simulink library "lib_rfsoc_fec"  (R2020b)
settings: Solver=VariableStepAuto  StartTime=0.0  StopTime=10.0  RelTol=1e-3
undefined symbols (not defined in the file): d, fs, generator_polynomial
libraries: commseqgen3 x84, hdlsllib x83, $bdroot x33, simulink x22, dspsigops x13
(part 4 of 4)

== system lib_rfsoc_fec/QAM Mapping/QAM Mapping/N-Width QAM-16 Symbol Mapping Real/QAM-16 Symbol Mapping 0 ==
  bits : Inport
  Bit Slice2 : hdlsllib/Logic and Bit Operations/Bit Slice  lidx=n+3  ridx=n+2
      settings: SourceProductBaseCode=SL
  Constant1 : Constant  Value=3  OutDataTypeStr=fixdt(1,3,0)  SampleTime=-1
  Constant2 : Constant  OutDataTypeStr=fixdt(1,3,0)  SampleTime=-1
  Constant3 : Constant  Value=-1  OutDataTypeStr=fixdt(1,3,0)  SampleTime=-1
  Constant4 : Constant  Value=-3  OutDataTypeStr=fixdt(1,3,0)  SampleTime=-1
  Multiport Switch : MultiPortSwitch  DataPortOrder=Zero-based contiguous  Inputs=4  zeroidx=on
  I : Outport
  wires:
  Multiport Switch/1 -> I/1
  Constant2/1 -> Multiport Switch/5
  Constant1/1 -> Multiport Switch/4
  Constant4/1 -> Multiport Switch/2
  Constant3/1 -> Multiport Switch/3
  bits/1 -> Bit Slice2/1
  Bit Slice2/1 -> Multiport Switch/1

== system lib_rfsoc_fec/QAM Mapping/QAM Mapping/N-Width QAM-16 Symbol Mapping Real/QAM-16 Symbol Mapping 1 ==
  bits : Inport
  Bit Slice2 : hdlsllib/Logic and Bit Operations/Bit Slice  lidx=n+3  ridx=n+2
      settings: SourceProductBaseCode=SL
  Constant1 : Constant  Value=3  OutDataTypeStr=fixdt(1,3,0)  SampleTime=-1
  Constant2 : Constant  OutDataTypeStr=fixdt(1,3,0)  SampleTime=-1
  Constant3 : Constant  Value=-1  OutDataTypeStr=fixdt(1,3,0)  SampleTime=-1
  Constant4 : Constant  Value=-3  OutDataTypeStr=fixdt(1,3,0)  SampleTime=-1
  Multiport Switch : MultiPortSwitch  DataPortOrder=Zero-based contiguous  Inputs=4  zeroidx=on
  I : Outport
  wires:
  Bit Slice2/1 -> Multiport Switch/1
  bits/1 -> Bit Slice2/1
  Constant3/1 -> Multiport Switch/3
  Constant4/1 -> Multiport Switch/2
  Constant1/1 -> Multiport Switch/4
  Constant2/1 -> Multiport Switch/5
  Multiport Switch/1 -> I/1

== system lib_rfsoc_fec/QAM Mapping/QAM Mapping/N-Width QAM-16 Symbol Mapping Real/QAM-16 Symbol Mapping 10 ==
  bits : Inport
  Bit Slice2 : hdlsllib/Logic and Bit Operations/Bit Slice  lidx=n+3  ridx=n+2
      settings: SourceProductBaseCode=SL
  Constant1 : Constant  Value=3  OutDataTypeStr=fixdt(1,3,0)  SampleTime=-1
  Constant2 : Constant  OutDataTypeStr=fixdt(1,3,0)  SampleTime=-1
  Constant3 : Constant  Value=-1  OutDataTypeStr=fixdt(1,3,0)  SampleTime=-1
  Constant4 : Constant  Value=-3  OutDataTypeStr=fixdt(1,3,0)  SampleTime=-1
  Multiport Switch : MultiPortSwitch  DataPortOrder=Zero-based contiguous  Inputs=4  zeroidx=on
  I : Outport
  wires:
  Bit Slice2/1 -> Multiport Switch/1
  bits/1 -> Bit Slice2/1
  Constant3/1 -> Multiport Switch/3
  Constant4/1 -> Multiport Switch/2
  Constant1/1 -> Multiport Switch/4
  Constant2/1 -> Multiport Switch/5
  Multiport Switch/1 -> I/1

== system lib_rfsoc_fec/QAM Mapping/QAM Mapping/N-Width QAM-16 Symbol Mapping Real/QAM-16 Symbol Mapping 11 ==
  bits : Inport
  Bit Slice2 : hdlsllib/Logic and Bit Operations/Bit Slice  lidx=n+3  ridx=n+2
      settings: SourceProductBaseCode=SL
  Constant1 : Constant  Value=3  OutDataTypeStr=fixdt(1,3,0)  SampleTime=-1
  Constant2 : Constant  OutDataTypeStr=fixdt(1,3,0)  SampleTime=-1
  Constant3 : Constant  Value=-1  OutDataTypeStr=fixdt(1,3,0)  SampleTime=-1
  Constant4 : Constant  Value=-3  OutDataTypeStr=fixdt(1,3,0)  SampleTime=-1
  Multiport Switch : MultiPortSwitch  DataPortOrder=Zero-based contiguous  Inputs=4  zeroidx=on
  I : Outport
  wires:
  Bit Slice2/1 -> Multiport Switch/1
  bits/1 -> Bit Slice2/1
  Constant3/1 -> Multiport Switch/3
  Constant4/1 -> Multiport Switch/2
  Constant1/1 -> Multiport Switch/4
  Constant2/1 -> Multiport Switch/5
  Multiport Switch/1 -> I/1

== system lib_rfsoc_fec/QAM Mapping/QAM Mapping/N-Width QAM-16 Symbol Mapping Real/QAM-16 Symbol Mapping 12 ==
  bits : Inport
  Bit Slice2 : hdlsllib/Logic and Bit Operations/Bit Slice  lidx=n+3  ridx=n+2
      settings: SourceProductBaseCode=SL
  Constant1 : Constant  Value=3  OutDataTypeStr=fixdt(1,3,0)  SampleTime=-1
  Constant2 : Constant  OutDataTypeStr=fixdt(1,3,0)  SampleTime=-1
  Constant3 : Constant  Value=-1  OutDataTypeStr=fixdt(1,3,0)  SampleTime=-1
  Constant4 : Constant  Value=-3  OutDataTypeStr=fixdt(1,3,0)  SampleTime=-1
  Multiport Switch : MultiPortSwitch  DataPortOrder=Zero-based contiguous  Inputs=4  zeroidx=on
  I : Outport
  wires:
  Bit Slice2/1 -> Multiport Switch/1
  bits/1 -> Bit Slice2/1
  Constant3/1 -> Multiport Switch/3
  Constant4/1 -> Multiport Switch/2
  Constant1/1 -> Multiport Switch/4
  Constant2/1 -> Multiport Switch/5
  Multiport Switch/1 -> I/1

== system lib_rfsoc_fec/QAM Mapping/QAM Mapping/N-Width QAM-16 Symbol Mapping Real/QAM-16 Symbol Mapping 13 ==
  bits : Inport
  Bit Slice2 : hdlsllib/Logic and Bit Operations/Bit Slice  lidx=n+3  ridx=n+2
      settings: SourceProductBaseCode=SL
  Constant1 : Constant  Value=3  OutDataTypeStr=fixdt(1,3,0)  SampleTime=-1
  Constant2 : Constant  OutDataTypeStr=fixdt(1,3,0)  SampleTime=-1
  Constant3 : Constant  Value=-1  OutDataTypeStr=fixdt(1,3,0)  SampleTime=-1
  Constant4 : Constant  Value=-3  OutDataTypeStr=fixdt(1,3,0)  SampleTime=-1
  Multiport Switch : MultiPortSwitch  DataPortOrder=Zero-based contiguous  Inputs=4  zeroidx=on
  I : Outport
  wires:
  Bit Slice2/1 -> Multiport Switch/1
  bits/1 -> Bit Slice2/1
  Constant3/1 -> Multiport Switch/3
  Constant4/1 -> Multiport Switch/2
  Constant1/1 -> Multiport Switch/4
  Constant2/1 -> Multiport Switch/5
  Multiport Switch/1 -> I/1

== system lib_rfsoc_fec/QAM Mapping/QAM Mapping/N-Width QAM-16 Symbol Mapping Real/QAM-16 Symbol Mapping 14 ==
  bits : Inport
  Bit Slice2 : hdlsllib/Logic and Bit Operations/Bit Slice  lidx=n+3  ridx=n+2
      settings: SourceProductBaseCode=SL
  Constant1 : Constant  Value=3  OutDataTypeStr=fixdt(1,3,0)  SampleTime=-1
  Constant2 : Constant  OutDataTypeStr=fixdt(1,3,0)  SampleTime=-1
  Constant3 : Constant  Value=-1  OutDataTypeStr=fixdt(1,3,0)  SampleTime=-1
  Constant4 : Constant  Value=-3  OutDataTypeStr=fixdt(1,3,0)  SampleTime=-1
  Multiport Switch : MultiPortSwitch  DataPortOrder=Zero-based contiguous  Inputs=4  zeroidx=on
  I : Outport
  wires:
  Bit Slice2/1 -> Multiport Switch/1
  bits/1 -> Bit Slice2/1
  Constant3/1 -> Multiport Switch/3
  Constant4/1 -> Multiport Switch/2
  Constant1/1 -> Multiport Switch/4
  Constant2/1 -> Multiport Switch/5
  Multiport Switch/1 -> I/1

== system lib_rfsoc_fec/QAM Mapping/QAM Mapping/N-Width QAM-16 Symbol Mapping Real/QAM-16 Symbol Mapping 15 ==
  bits : Inport
  Bit Slice2 : hdlsllib/Logic and Bit Operations/Bit Slice  lidx=n+3  ridx=n+2
      settings: SourceProductBaseCode=SL
  Constant1 : Constant  Value=3  OutDataTypeStr=fixdt(1,3,0)  SampleTime=-1
  Constant2 : Constant  OutDataTypeStr=fixdt(1,3,0)  SampleTime=-1
  Constant3 : Constant  Value=-1  OutDataTypeStr=fixdt(1,3,0)  SampleTime=-1
  Constant4 : Constant  Value=-3  OutDataTypeStr=fixdt(1,3,0)  SampleTime=-1
  Multiport Switch : MultiPortSwitch  DataPortOrder=Zero-based contiguous  Inputs=4  zeroidx=on
  I : Outport
  wires:
  Bit Slice2/1 -> Multiport Switch/1
  bits/1 -> Bit Slice2/1
  Constant3/1 -> Multiport Switch/3
  Constant4/1 -> Multiport Switch/2
  Constant1/1 -> Multiport Switch/4
  Constant2/1 -> Multiport Switch/5
  Multiport Switch/1 -> I/1

== system lib_rfsoc_fec/QAM Mapping/QAM Mapping/N-Width QAM-16 Symbol Mapping Real/QAM-16 Symbol Mapping 16 ==
  bits : Inport
  Bit Slice2 : hdlsllib/Logic and Bit Operations/Bit Slice  lidx=n+3  ridx=n+2
      settings: SourceProductBaseCode=SL
  Constant1 : Constant  Value=3  OutDataTypeStr=fixdt(1,3,0)  SampleTime=-1
  Constant2 : Constant  OutDataTypeStr=fixdt(1,3,0)  SampleTime=-1
  Constant3 : Constant  Value=-1  OutDataTypeStr=fixdt(1,3,0)  SampleTime=-1
  Constant4 : Constant  Value=-3  OutDataTypeStr=fixdt(1,3,0)  SampleTime=-1
  Multiport Switch : MultiPortSwitch  DataPortOrder=Zero-based contiguous  Inputs=4  zeroidx=on
  I : Outport
  wires:
  Bit Slice2/1 -> Multiport Switch/1
  bits/1 -> Bit Slice2/1
  Constant3/1 -> Multiport Switch/3
  Constant4/1 -> Multiport Switch/2
  Constant1/1 -> Multiport Switch/4
  Constant2/1 -> Multiport Switch/5
  Multiport Switch/1 -> I/1

== system lib_rfsoc_fec/QAM Mapping/QAM Mapping/N-Width QAM-16 Symbol Mapping Real/QAM-16 Symbol Mapping 17 ==
  bits : Inport
  Bit Slice2 : hdlsllib/Logic and Bit Operations/Bit Slice  lidx=n+3  ridx=n+2
      settings: SourceProductBaseCode=SL
  Constant1 : Constant  Value=3  OutDataTypeStr=fixdt(1,3,0)  SampleTime=-1
  Constant2 : Constant  OutDataTypeStr=fixdt(1,3,0)  SampleTime=-1
  Constant3 : Constant  Value=-1  OutDataTypeStr=fixdt(1,3,0)  SampleTime=-1
  Constant4 : Constant  Value=-3  OutDataTypeStr=fixdt(1,3,0)  SampleTime=-1
  Multiport Switch : MultiPortSwitch  DataPortOrder=Zero-based contiguous  Inputs=4  zeroidx=on
  I : Outport
  wires:
  Bit Slice2/1 -> Multiport Switch/1
  bits/1 -> Bit Slice2/1
  Constant3/1 -> Multiport Switch/3
  Constant4/1 -> Multiport Switch/2
  Constant1/1 -> Multiport Switch/4
  Constant2/1 -> Multiport Switch/5
  Multiport Switch/1 -> I/1

== system lib_rfsoc_fec/QAM Mapping/QAM Mapping/N-Width QAM-16 Symbol Mapping Real/QAM-16 Symbol Mapping 18 ==
  bits : Inport
  Bit Slice2 : hdlsllib/Logic and Bit Operations/Bit Slice  lidx=n+3  ridx=n+2
      settings: SourceProductBaseCode=SL
  Constant1 : Constant  Value=3  OutDataTypeStr=fixdt(1,3,0)  SampleTime=-1
  Constant2 : Constant  OutDataTypeStr=fixdt(1,3,0)  SampleTime=-1
  Constant3 : Constant  Value=-1  OutDataTypeStr=fixdt(1,3,0)  SampleTime=-1
  Constant4 : Constant  Value=-3  OutDataTypeStr=fixdt(1,3,0)  SampleTime=-1
  Multiport Switch : MultiPortSwitch  DataPortOrder=Zero-based contiguous  Inputs=4  zeroidx=on
  I : Outport
  wires:
  Bit Slice2/1 -> Multiport Switch/1
  bits/1 -> Bit Slice2/1
  Constant3/1 -> Multiport Switch/3
  Constant4/1 -> Multiport Switch/2
  Constant1/1 -> Multiport Switch/4
  Constant2/1 -> Multiport Switch/5
  Multiport Switch/1 -> I/1

== system lib_rfsoc_fec/QAM Mapping/QAM Mapping/N-Width QAM-16 Symbol Mapping Real/QAM-16 Symbol Mapping 19 ==
  bits : Inport
  Bit Slice2 : hdlsllib/Logic and Bit Operations/Bit Slice  lidx=n+3  ridx=n+2
      settings: SourceProductBaseCode=SL
  Constant1 : Constant  Value=3  OutDataTypeStr=fixdt(1,3,0)  SampleTime=-1
  Constant2 : Constant  OutDataTypeStr=fixdt(1,3,0)  SampleTime=-1
  Constant3 : Constant  Value=-1  OutDataTypeStr=fixdt(1,3,0)  SampleTime=-1
  Constant4 : Constant  Value=-3  OutDataTypeStr=fixdt(1,3,0)  SampleTime=-1
  Multiport Switch : MultiPortSwitch  DataPortOrder=Zero-based contiguous  Inputs=4  zeroidx=on
  I : Outport
  wires:
  Bit Slice2/1 -> Multiport Switch/1
  bits/1 -> Bit Slice2/1
  Constant3/1 -> Multiport Switch/3
  Constant4/1 -> Multiport Switch/2
  Constant1/1 -> Multiport Switch/4
  Constant2/1 -> Multiport Switch/5
  Multiport Switch/1 -> I/1

== system lib_rfsoc_fec/QAM Mapping/QAM Mapping/N-Width QAM-16 Symbol Mapping Real/QAM-16 Symbol Mapping 2 ==
  bits : Inport
  Bit Slice2 : hdlsllib/Logic and Bit Operations/Bit Slice  lidx=n+3  ridx=n+2
      settings: SourceProductBaseCode=SL
  Constant1 : Constant  Value=3  OutDataTypeStr=fixdt(1,3,0)  SampleTime=-1
  Constant2 : Constant  OutDataTypeStr=fixdt(1,3,0)  SampleTime=-1
  Constant3 : Constant  Value=-1  OutDataTypeStr=fixdt(1,3,0)  SampleTime=-1
  Constant4 : Constant  Value=-3  OutDataTypeStr=fixdt(1,3,0)  SampleTime=-1
  Multiport Switch : MultiPortSwitch  DataPortOrder=Zero-based contiguous  Inputs=4  zeroidx=on
  I : Outport
  wires:
  Bit Slice2/1 -> Multiport Switch/1
  bits/1 -> Bit Slice2/1
  Constant3/1 -> Multiport Switch/3
  Constant4/1 -> Multiport Switch/2
  Constant1/1 -> Multiport Switch/4
  Constant2/1 -> Multiport Switch/5
  Multiport Switch/1 -> I/1

== system lib_rfsoc_fec/QAM Mapping/QAM Mapping/N-Width QAM-16 Symbol Mapping Real/QAM-16 Symbol Mapping 20 ==
  bits : Inport
  Bit Slice2 : hdlsllib/Logic and Bit Operations/Bit Slice  lidx=n+3  ridx=n+2
      settings: SourceProductBaseCode=SL
  Constant1 : Constant  Value=3  OutDataTypeStr=fixdt(1,3,0)  SampleTime=-1
  Constant2 : Constant  OutDataTypeStr=fixdt(1,3,0)  SampleTime=-1
  Constant3 : Constant  Value=-1  OutDataTypeStr=fixdt(1,3,0)  SampleTime=-1
  Constant4 : Constant  Value=-3  OutDataTypeStr=fixdt(1,3,0)  SampleTime=-1
  Multiport Switch : MultiPortSwitch  DataPortOrder=Zero-based contiguous  Inputs=4  zeroidx=on
  I : Outport
  wires:
  Bit Slice2/1 -> Multiport Switch/1
  bits/1 -> Bit Slice2/1
  Constant3/1 -> Multiport Switch/3
  Constant4/1 -> Multiport Switch/2
  Constant1/1 -> Multiport Switch/4
  Constant2/1 -> Multiport Switch/5
  Multiport Switch/1 -> I/1

== system lib_rfsoc_fec/QAM Mapping/QAM Mapping/N-Width QAM-16 Symbol Mapping Real/QAM-16 Symbol Mapping 21 ==
  bits : Inport
  Bit Slice2 : hdlsllib/Logic and Bit Operations/Bit Slice  lidx=n+3  ridx=n+2
      settings: SourceProductBaseCode=SL
  Constant1 : Constant  Value=3  OutDataTypeStr=fixdt(1,3,0)  SampleTime=-1
  Constant2 : Constant  OutDataTypeStr=fixdt(1,3,0)  SampleTime=-1
  Constant3 : Constant  Value=-1  OutDataTypeStr=fixdt(1,3,0)  SampleTime=-1
  Constant4 : Constant  Value=-3  OutDataTypeStr=fixdt(1,3,0)  SampleTime=-1
  Multiport Switch : MultiPortSwitch  DataPortOrder=Zero-based contiguous  Inputs=4  zeroidx=on
  I : Outport
  wires:
  Bit Slice2/1 -> Multiport Switch/1
  bits/1 -> Bit Slice2/1
  Constant3/1 -> Multiport Switch/3
  Constant4/1 -> Multiport Switch/2
  Constant1/1 -> Multiport Switch/4
  Constant2/1 -> Multiport Switch/5
  Multiport Switch/1 -> I/1

== system lib_rfsoc_fec/QAM Mapping/QAM Mapping/N-Width QAM-16 Symbol Mapping Real/QAM-16 Symbol Mapping 22 ==
  bits : Inport
  Bit Slice2 : hdlsllib/Logic and Bit Operations/Bit Slice  lidx=n+3  ridx=n+2
      settings: SourceProductBaseCode=SL
  Constant1 : Constant  Value=3  OutDataTypeStr=fixdt(1,3,0)  SampleTime=-1
  Constant2 : Constant  OutDataTypeStr=fixdt(1,3,0)  SampleTime=-1
  Constant3 : Constant  Value=-1  OutDataTypeStr=fixdt(1,3,0)  SampleTime=-1
  Constant4 : Constant  Value=-3  OutDataTypeStr=fixdt(1,3,0)  SampleTime=-1
  Multiport Switch : MultiPortSwitch  DataPortOrder=Zero-based contiguous  Inputs=4  zeroidx=on
  I : Outport
  wires:
  Bit Slice2/1 -> Multiport Switch/1
  bits/1 -> Bit Slice2/1
  Constant3/1 -> Multiport Switch/3
  Constant4/1 -> Multiport Switch/2
  Constant1/1 -> Multiport Switch/4
  Constant2/1 -> Multiport Switch/5
  Multiport Switch/1 -> I/1

== system lib_rfsoc_fec/QAM Mapping/QAM Mapping/N-Width QAM-16 Symbol Mapping Real/QAM-16 Symbol Mapping 23 ==
  bits : Inport
  Bit Slice2 : hdlsllib/Logic and Bit Operations/Bit Slice  lidx=n+3  ridx=n+2
      settings: SourceProductBaseCode=SL
  Constant1 : Constant  Value=3  OutDataTypeStr=fixdt(1,3,0)  SampleTime=-1
  Constant2 : Constant  OutDataTypeStr=fixdt(1,3,0)  SampleTime=-1
  Constant3 : Constant  Value=-1  OutDataTypeStr=fixdt(1,3,0)  SampleTime=-1
  Constant4 : Constant  Value=-3  OutDataTypeStr=fixdt(1,3,0)  SampleTime=-1
  Multiport Switch : MultiPortSwitch  DataPortOrder=Zero-based contiguous  Inputs=4  zeroidx=on
  I : Outport
  wires:
  Bit Slice2/1 -> Multiport Switch/1
  bits/1 -> Bit Slice2/1
  Constant3/1 -> Multiport Switch/3
  Constant4/1 -> Multiport Switch/2
  Constant1/1 -> Multiport Switch/4
  Constant2/1 -> Multiport Switch/5
  Multiport Switch/1 -> I/1

== system lib_rfsoc_fec/QAM Mapping/QAM Mapping/N-Width QAM-16 Symbol Mapping Real/QAM-16 Symbol Mapping 24 ==
  bits : Inport
  Bit Slice2 : hdlsllib/Logic and Bit Operations/Bit Slice  lidx=n+3  ridx=n+2
      settings: SourceProductBaseCode=SL
  Constant1 : Constant  Value=3  OutDataTypeStr=fixdt(1,3,0)  SampleTime=-1
  Constant2 : Constant  OutDataTypeStr=fixdt(1,3,0)  SampleTime=-1
  Constant3 : Constant  Value=-1  OutDataTypeStr=fixdt(1,3,0)  SampleTime=-1
  Constant4 : Constant  Value=-3  OutDataTypeStr=fixdt(1,3,0)  SampleTime=-1
  Multiport Switch : MultiPortSwitch  DataPortOrder=Zero-based contiguous  Inputs=4  zeroidx=on
  I : Outport
  wires:
  Bit Slice2/1 -> Multiport Switch/1
  bits/1 -> Bit Slice2/1
  Constant3/1 -> Multiport Switch/3
  Constant4/1 -> Multiport Switch/2
  Constant1/1 -> Multiport Switch/4
  Constant2/1 -> Multiport Switch/5
  Multiport Switch/1 -> I/1

== system lib_rfsoc_fec/QAM Mapping/QAM Mapping/N-Width QAM-16 Symbol Mapping Real/QAM-16 Symbol Mapping 25 ==
  bits : Inport
  Bit Slice2 : hdlsllib/Logic and Bit Operations/Bit Slice  lidx=n+3  ridx=n+2
      settings: SourceProductBaseCode=SL
  Constant1 : Constant  Value=3  OutDataTypeStr=fixdt(1,3,0)  SampleTime=-1
  Constant2 : Constant  OutDataTypeStr=fixdt(1,3,0)  SampleTime=-1
  Constant3 : Constant  Value=-1  OutDataTypeStr=fixdt(1,3,0)  SampleTime=-1
  Constant4 : Constant  Value=-3  OutDataTypeStr=fixdt(1,3,0)  SampleTime=-1
  Multiport Switch : MultiPortSwitch  DataPortOrder=Zero-based contiguous  Inputs=4  zeroidx=on
  I : Outport
  wires:
  Bit Slice2/1 -> Multiport Switch/1
  bits/1 -> Bit Slice2/1
  Constant3/1 -> Multiport Switch/3
  Constant4/1 -> Multiport Switch/2
  Constant1/1 -> Multiport Switch/4
  Constant2/1 -> Multiport Switch/5
  Multiport Switch/1 -> I/1

== system lib_rfsoc_fec/QAM Mapping/QAM Mapping/N-Width QAM-16 Symbol Mapping Real/QAM-16 Symbol Mapping 26 ==
  bits : Inport
  Bit Slice2 : hdlsllib/Logic and Bit Operations/Bit Slice  lidx=n+3  ridx=n+2
      settings: SourceProductBaseCode=SL
  Constant1 : Constant  Value=3  OutDataTypeStr=fixdt(1,3,0)  SampleTime=-1
  Constant2 : Constant  OutDataTypeStr=fixdt(1,3,0)  SampleTime=-1
  Constant3 : Constant  Value=-1  OutDataTypeStr=fixdt(1,3,0)  SampleTime=-1
  Constant4 : Constant  Value=-3  OutDataTypeStr=fixdt(1,3,0)  SampleTime=-1
  Multiport Switch : MultiPortSwitch  DataPortOrder=Zero-based contiguous  Inputs=4  zeroidx=on
  I : Outport
  wires:
  Bit Slice2/1 -> Multiport Switch/1
  bits/1 -> Bit Slice2/1
  Constant3/1 -> Multiport Switch/3
  Constant4/1 -> Multiport Switch/2
  Constant1/1 -> Multiport Switch/4
  Constant2/1 -> Multiport Switch/5
  Multiport Switch/1 -> I/1

== system lib_rfsoc_fec/QAM Mapping/QAM Mapping/N-Width QAM-16 Symbol Mapping Real/QAM-16 Symbol Mapping 27 ==
  bits : Inport
  Bit Slice2 : hdlsllib/Logic and Bit Operations/Bit Slice  lidx=n+3  ridx=n+2
      settings: SourceProductBaseCode=SL
  Constant1 : Constant  Value=3  OutDataTypeStr=fixdt(1,3,0)  SampleTime=-1
  Constant2 : Constant  OutDataTypeStr=fixdt(1,3,0)  SampleTime=-1
  Constant3 : Constant  Value=-1  OutDataTypeStr=fixdt(1,3,0)  SampleTime=-1
  Constant4 : Constant  Value=-3  OutDataTypeStr=fixdt(1,3,0)  SampleTime=-1
  Multiport Switch : MultiPortSwitch  DataPortOrder=Zero-based contiguous  Inputs=4  zeroidx=on
  I : Outport
  wires:
  Bit Slice2/1 -> Multiport Switch/1
  bits/1 -> Bit Slice2/1
  Constant3/1 -> Multiport Switch/3
  Constant4/1 -> Multiport Switch/2
  Constant1/1 -> Multiport Switch/4
  Constant2/1 -> Multiport Switch/5
  Multiport Switch/1 -> I/1

== system lib_rfsoc_fec/QAM Mapping/QAM Mapping/N-Width QAM-16 Symbol Mapping Real/QAM-16 Symbol Mapping 28 ==
  bits : Inport
  Bit Slice2 : hdlsllib/Logic and Bit Operations/Bit Slice  lidx=n+3  ridx=n+2
      settings: SourceProductBaseCode=SL
  Constant1 : Constant  Value=3  OutDataTypeStr=fixdt(1,3,0)  SampleTime=-1
  Constant2 : Constant  OutDataTypeStr=fixdt(1,3,0)  SampleTime=-1
  Constant3 : Constant  Value=-1  OutDataTypeStr=fixdt(1,3,0)  SampleTime=-1
  Constant4 : Constant  Value=-3  OutDataTypeStr=fixdt(1,3,0)  SampleTime=-1
  Multiport Switch : MultiPortSwitch  DataPortOrder=Zero-based contiguous  Inputs=4  zeroidx=on
  I : Outport
  wires:
  Bit Slice2/1 -> Multiport Switch/1
  bits/1 -> Bit Slice2/1
  Constant3/1 -> Multiport Switch/3
  Constant4/1 -> Multiport Switch/2
  Constant1/1 -> Multiport Switch/4
  Constant2/1 -> Multiport Switch/5
  Multiport Switch/1 -> I/1

== system lib_rfsoc_fec/QAM Mapping/QAM Mapping/N-Width QAM-16 Symbol Mapping Real/QAM-16 Symbol Mapping 29 ==
  bits : Inport
  Bit Slice2 : hdlsllib/Logic and Bit Operations/Bit Slice  lidx=n+3  ridx=n+2
      settings: SourceProductBaseCode=SL
  Constant1 : Constant  Value=3  OutDataTypeStr=fixdt(1,3,0)  SampleTime=-1
  Constant2 : Constant  OutDataTypeStr=fixdt(1,3,0)  SampleTime=-1
  Constant3 : Constant  Value=-1  OutDataTypeStr=fixdt(1,3,0)  SampleTime=-1
  Constant4 : Constant  Value=-3  OutDataTypeStr=fixdt(1,3,0)  SampleTime=-1
  Multiport Switch : MultiPortSwitch  DataPortOrder=Zero-based contiguous  Inputs=4  zeroidx=on
  I : Outport
  wires:
  Bit Slice2/1 -> Multiport Switch/1
  bits/1 -> Bit Slice2/1
  Constant3/1 -> Multiport Switch/3
  Constant4/1 -> Multiport Switch/2
  Constant1/1 -> Multiport Switch/4
  Constant2/1 -> Multiport Switch/5
  Multiport Switch/1 -> I/1

== system lib_rfsoc_fec/QAM Mapping/QAM Mapping/N-Width QAM-16 Symbol Mapping Real/QAM-16 Symbol Mapping 3 ==
  bits : Inport
  Bit Slice2 : hdlsllib/Logic and Bit Operations/Bit Slice  lidx=n+3  ridx=n+2
      settings: SourceProductBaseCode=SL
  Constant1 : Constant  Value=3  OutDataTypeStr=fixdt(1,3,0)  SampleTime=-1
  Constant2 : Constant  OutDataTypeStr=fixdt(1,3,0)  SampleTime=-1
  Constant3 : Constant  Value=-1  OutDataTypeStr=fixdt(1,3,0)  SampleTime=-1
  Constant4 : Constant  Value=-3  OutDataTypeStr=fixdt(1,3,0)  SampleTime=-1
  Multiport Switch : MultiPortSwitch  DataPortOrder=Zero-based contiguous  Inputs=4  zeroidx=on
  I : Outport
  wires:
  Bit Slice2/1 -> Multiport Switch/1
  bits/1 -> Bit Slice2/1
  Constant3/1 -> Multiport Switch/3
  Constant4/1 -> Multiport Switch/2
  Constant1/1 -> Multiport Switch/4
  Constant2/1 -> Multiport Switch/5
  Multiport Switch/1 -> I/1

== system lib_rfsoc_fec/QAM Mapping/QAM Mapping/N-Width QAM-16 Symbol Mapping Real/QAM-16 Symbol Mapping 30 ==
  bits : Inport
  Bit Slice2 : hdlsllib/Logic and Bit Operations/Bit Slice  lidx=n+3  ridx=n+2
      settings: SourceProductBaseCode=SL
  Constant1 : Constant  Value=3  OutDataTypeStr=fixdt(1,3,0)  SampleTime=-1
  Constant2 : Constant  OutDataTypeStr=fixdt(1,3,0)  SampleTime=-1
  Constant3 : Constant  Value=-1  OutDataTypeStr=fixdt(1,3,0)  SampleTime=-1
  Constant4 : Constant  Value=-3  OutDataTypeStr=fixdt(1,3,0)  SampleTime=-1
  Multiport Switch : MultiPortSwitch  DataPortOrder=Zero-based contiguous  Inputs=4  zeroidx=on
  I : Outport
  wires:
  Bit Slice2/1 -> Multiport Switch/1
  bits/1 -> Bit Slice2/1
  Constant3/1 -> Multiport Switch/3
  Constant4/1 -> Multiport Switch/2
  Constant1/1 -> Multiport Switch/4
  Constant2/1 -> Multiport Switch/5
  Multiport Switch/1 -> I/1

== system lib_rfsoc_fec/QAM Mapping/QAM Mapping/N-Width QAM-16 Symbol Mapping Real/QAM-16 Symbol Mapping 31 ==
  bits : Inport
  Bit Slice2 : hdlsllib/Logic and Bit Operations/Bit Slice  lidx=n+3  ridx=n+2
      settings: SourceProductBaseCode=SL
  Constant1 : Constant  Value=3  OutDataTypeStr=fixdt(1,3,0)  SampleTime=-1
  Constant2 : Constant  OutDataTypeStr=fixdt(1,3,0)  SampleTime=-1
  Constant3 : Constant  Value=-1  OutDataTypeStr=fixdt(1,3,0)  SampleTime=-1
  Constant4 : Constant  Value=-3  OutDataTypeStr=fixdt(1,3,0)  SampleTime=-1
  Multiport Switch : MultiPortSwitch  DataPortOrder=Zero-based contiguous  Inputs=4  zeroidx=on
  I : Outport
  wires:
  Bit Slice2/1 -> Multiport Switch/1
  bits/1 -> Bit Slice2/1
  Constant3/1 -> Multiport Switch/3
  Constant4/1 -> Multiport Switch/2
  Constant1/1 -> Multiport Switch/4
  Constant2/1 -> Multiport Switch/5
  Multiport Switch/1 -> I/1

== system lib_rfsoc_fec/QAM Mapping/QAM Mapping/N-Width QAM-16 Symbol Mapping Real/QAM-16 Symbol Mapping 4 ==
  bits : Inport
  Bit Slice2 : hdlsllib/Logic and Bit Operations/Bit Slice  lidx=n+3  ridx=n+2
      settings: SourceProductBaseCode=SL
  Constant1 : Constant  Value=3  OutDataTypeStr=fixdt(1,3,0)  SampleTime=-1
  Constant2 : Constant  OutDataTypeStr=fixdt(1,3,0)  SampleTime=-1
  Constant3 : Constant  Value=-1  OutDataTypeStr=fixdt(1,3,0)  SampleTime=-1
  Constant4 : Constant  Value=-3  OutDataTypeStr=fixdt(1,3,0)  SampleTime=-1
  Multiport Switch : MultiPortSwitch  DataPortOrder=Zero-based contiguous  Inputs=4  zeroidx=on
  I : Outport
  wires:
  Bit Slice2/1 -> Multiport Switch/1
  bits/1 -> Bit Slice2/1
  Constant3/1 -> Multiport Switch/3
  Constant4/1 -> Multiport Switch/2
  Constant1/1 -> Multiport Switch/4
  Constant2/1 -> Multiport Switch/5
  Multiport Switch/1 -> I/1

== system lib_rfsoc_fec/QAM Mapping/QAM Mapping/N-Width QAM-16 Symbol Mapping Real/QAM-16 Symbol Mapping 5 ==
  bits : Inport
  Bit Slice2 : hdlsllib/Logic and Bit Operations/Bit Slice  lidx=n+3  ridx=n+2
      settings: SourceProductBaseCode=SL
  Constant1 : Constant  Value=3  OutDataTypeStr=fixdt(1,3,0)  SampleTime=-1
  Constant2 : Constant  OutDataTypeStr=fixdt(1,3,0)  SampleTime=-1
  Constant3 : Constant  Value=-1  OutDataTypeStr=fixdt(1,3,0)  SampleTime=-1
  Constant4 : Constant  Value=-3  OutDataTypeStr=fixdt(1,3,0)  SampleTime=-1
  Multiport Switch : MultiPortSwitch  DataPortOrder=Zero-based contiguous  Inputs=4  zeroidx=on
  I : Outport
  wires:
  Bit Slice2/1 -> Multiport Switch/1
  bits/1 -> Bit Slice2/1
  Constant3/1 -> Multiport Switch/3
  Constant4/1 -> Multiport Switch/2
  Constant1/1 -> Multiport Switch/4
  Constant2/1 -> Multiport Switch/5
  Multiport Switch/1 -> I/1

== system lib_rfsoc_fec/QAM Mapping/QAM Mapping/N-Width QAM-16 Symbol Mapping Real/QAM-16 Symbol Mapping 6 ==
  bits : Inport
  Bit Slice2 : hdlsllib/Logic and Bit Operations/Bit Slice  lidx=n+3  ridx=n+2
      settings: SourceProductBaseCode=SL
  Constant1 : Constant  Value=3  OutDataTypeStr=fixdt(1,3,0)  SampleTime=-1
  Constant2 : Constant  OutDataTypeStr=fixdt(1,3,0)  SampleTime=-1
  Constant3 : Constant  Value=-1  OutDataTypeStr=fixdt(1,3,0)  SampleTime=-1
  Constant4 : Constant  Value=-3  OutDataTypeStr=fixdt(1,3,0)  SampleTime=-1
  Multiport Switch : MultiPortSwitch  DataPortOrder=Zero-based contiguous  Inputs=4  zeroidx=on
  I : Outport
  wires:
  Bit Slice2/1 -> Multiport Switch/1
  bits/1 -> Bit Slice2/1
  Constant3/1 -> Multiport Switch/3
  Constant4/1 -> Multiport Switch/2
  Constant1/1 -> Multiport Switch/4
  Constant2/1 -> Multiport Switch/5
  Multiport Switch/1 -> I/1

== system lib_rfsoc_fec/QAM Mapping/QAM Mapping/N-Width QAM-16 Symbol Mapping Real/QAM-16 Symbol Mapping 7 ==
  bits : Inport
  Bit Slice2 : hdlsllib/Logic and Bit Operations/Bit Slice  lidx=n+3  ridx=n+2
      settings: SourceProductBaseCode=SL
  Constant1 : Constant  Value=3  OutDataTypeStr=fixdt(1,3,0)  SampleTime=-1
  Constant2 : Constant  OutDataTypeStr=fixdt(1,3,0)  SampleTime=-1
  Constant3 : Constant  Value=-1  OutDataTypeStr=fixdt(1,3,0)  SampleTime=-1
  Constant4 : Constant  Value=-3  OutDataTypeStr=fixdt(1,3,0)  SampleTime=-1
  Multiport Switch : MultiPortSwitch  DataPortOrder=Zero-based contiguous  Inputs=4  zeroidx=on
  I : Outport
  wires:
  Bit Slice2/1 -> Multiport Switch/1
  bits/1 -> Bit Slice2/1
  Constant3/1 -> Multiport Switch/3
  Constant4/1 -> Multiport Switch/2
  Constant1/1 -> Multiport Switch/4
  Constant2/1 -> Multiport Switch/5
  Multiport Switch/1 -> I/1

== system lib_rfsoc_fec/QAM Mapping/QAM Mapping/N-Width QAM-16 Symbol Mapping Real/QAM-16 Symbol Mapping 8 ==
  bits : Inport
  Bit Slice2 : hdlsllib/Logic and Bit Operations/Bit Slice  lidx=n+3  ridx=n+2
      settings: SourceProductBaseCode=SL
  Constant1 : Constant  Value=3  OutDataTypeStr=fixdt(1,3,0)  SampleTime=-1
  Constant2 : Constant  OutDataTypeStr=fixdt(1,3,0)  SampleTime=-1
  Constant3 : Constant  Value=-1  OutDataTypeStr=fixdt(1,3,0)  SampleTime=-1
  Constant4 : Constant  Value=-3  OutDataTypeStr=fixdt(1,3,0)  SampleTime=-1
  Multiport Switch : MultiPortSwitch  DataPortOrder=Zero-based contiguous  Inputs=4  zeroidx=on
  I : Outport
  wires:
  Bit Slice2/1 -> Multiport Switch/1
  bits/1 -> Bit Slice2/1
  Constant3/1 -> Multiport Switch/3
  Constant4/1 -> Multiport Switch/2
  Constant1/1 -> Multiport Switch/4
  Constant2/1 -> Multiport Switch/5
  Multiport Switch/1 -> I/1

== system lib_rfsoc_fec/QAM Mapping/QAM Mapping/N-Width QAM-16 Symbol Mapping Real/QAM-16 Symbol Mapping 9 ==
  bits : Inport
  Bit Slice2 : hdlsllib/Logic and Bit Operations/Bit Slice  lidx=n+3  ridx=n+2
      settings: SourceProductBaseCode=SL
  Constant1 : Constant  Value=3  OutDataTypeStr=fixdt(1,3,0)  SampleTime=-1
  Constant2 : Constant  OutDataTypeStr=fixdt(1,3,0)  SampleTime=-1
  Constant3 : Constant  Value=-1  OutDataTypeStr=fixdt(1,3,0)  SampleTime=-1
  Constant4 : Constant  Value=-3  OutDataTypeStr=fixdt(1,3,0)  SampleTime=-1
  Multiport Switch : MultiPortSwitch  DataPortOrder=Zero-based contiguous  Inputs=4  zeroidx=on
  I : Outport
  wires:
  Bit Slice2/1 -> Multiport Switch/1
  bits/1 -> Bit Slice2/1
  Constant3/1 -> Multiport Switch/3
  Constant4/1 -> Multiport Switch/2
  Constant1/1 -> Multiport Switch/4
  Constant2/1 -> Multiport Switch/5
  Multiport Switch/1 -> I/1

== system lib_rfsoc_fec/Random Number Generator/concat/mask_generator/falling_edge ==
  in : Inport
  Data Type Conversion1 : DataTypeConversion  OutDataTypeStr=boolean  SaturateOnIntegerOverflow=on  RndMeth=Zero
  Delay15 : Delay  DelayLength=1  InitialCondition=1  InputProcessing=Columns as channels (frame based)
  Logical Operator1 : Logic  Operator=NOT  Inputs=1
  Logical Operator3 : Logic
  pulse : Outport
  wires:
  Logical Operator3/1 -> pulse/1
  in/1 -> Data Type Conversion1/1
  Delay15/1 -> Logical Operator3/2
  Data Type Conversion1/1 -> Logical Operator1/1, Delay15/1
  Logical Operator1/1 -> Logical Operator3/1

== system lib_rfsoc_fec/Soft Demodulation/Soft Demodulation/Subsystem1/get_min1 ==
  a : Inport
  b : Inport  Port=2
  Compare To Zero : simulink/Logic and Bit Operations/Compare To Zero  relop=<=  OutDataTypeStr=boolean
  Multiport Switch2 : MultiPortSwitch  DataPortOrder=Zero-based contiguous  Inputs=2  zeroidx=on
  Subtract18 : Sum  Inputs=+-  OutDataTypeStr=fixdt(1,46,28)
  min : Outport
  wires:
  Compare To Zero/1 -> Multiport Switch2/1
  Multiport Switch2/1 -> min/1
  a/1 -> Subtract18/1, Multiport Switch2/3
  b/1 -> Multiport Switch2/2, Subtract18/2
  Subtract18/1 -> Compare To Zero/1

== system lib_rfsoc_fec/Soft Demodulation/Soft Demodulation/Subsystem1/get_min2 ==
  a : Inport
  b : Inport  Port=2
  Compare To Zero : simulink/Logic and Bit Operations/Compare To Zero  relop=<=  OutDataTypeStr=boolean
  Multiport Switch2 : MultiPortSwitch  DataPortOrder=Zero-based contiguous  Inputs=2  zeroidx=on
  Subtract18 : Sum  Inputs=+-  OutDataTypeStr=fixdt(1,46,28)
  min : Outport
  wires:
  Subtract18/1 -> Compare To Zero/1
  b/1 -> Subtract18/2, Multiport Switch2/2
  a/1 -> Multiport Switch2/3, Subtract18/1
  Multiport Switch2/1 -> min/1
  Compare To Zero/1 -> Multiport Switch2/1

== system lib_rfsoc_fec/Soft Demodulation/Soft Demodulation/Subsystem1/get_min3 ==
  a : Inport
  b : Inport  Port=2
  Compare To Zero : simulink/Logic and Bit Operations/Compare To Zero  relop=<=  OutDataTypeStr=boolean
  Multiport Switch2 : MultiPortSwitch  DataPortOrder=Zero-based contiguous  Inputs=2  zeroidx=on
  Subtract18 : Sum  Inputs=+-  OutDataTypeStr=fixdt(1,46,28)
  min : Outport
  wires:
  Compare To Zero/1 -> Multiport Switch2/1
  Multiport Switch2/1 -> min/1
  a/1 -> Subtract18/1, Multiport Switch2/3
  b/1 -> Multiport Switch2/2, Subtract18/2
  Subtract18/1 -> Compare To Zero/1

== system lib_rfsoc_fec/Soft Demodulation/Soft Demodulation/Subsystem1/get_min4 ==
  a : Inport
  b : Inport  Port=2
  Compare To Zero : simulink/Logic and Bit Operations/Compare To Zero  relop=<=  OutDataTypeStr=boolean
  Multiport Switch2 : MultiPortSwitch  DataPortOrder=Zero-based contiguous  Inputs=2  zeroidx=on
  Subtract18 : Sum  Inputs=+-  OutDataTypeStr=fixdt(1,46,28)
  min : Outport
  wires:
  Subtract18/1 -> Compare To Zero/1
  b/1 -> Subtract18/2, Multiport Switch2/2
  a/1 -> Multiport Switch2/3, Subtract18/1
  Multiport Switch2/1 -> min/1
  Compare To Zero/1 -> Multiport Switch2/1

== system lib_rfsoc_fec/Soft Demodulation/Soft Demodulation/Subsystem1/get_min5 ==
  a : Inport
  b : Inport  Port=2
  Compare To Zero : simulink/Logic and Bit Operations/Compare To Zero  relop=<=  OutDataTypeStr=boolean
  Multiport Switch2 : MultiPortSwitch  DataPortOrder=Zero-based contiguous  Inputs=2  zeroidx=on
  Subtract18 : Sum  Inputs=+-  OutDataTypeStr=fixdt(1,46,28)
  min : Outport
  wires:
  Compare To Zero/1 -> Multiport Switch2/1
  Multiport Switch2/1 -> min/1
  a/1 -> Subtract18/1, Multiport Switch2/3
  b/1 -> Multiport Switch2/2, Subtract18/2
  Subtract18/1 -> Compare To Zero/1

== system lib_rfsoc_fec/Soft Demodulation/Soft Demodulation/Subsystem1/get_min6 ==
  a : Inport
  b : Inport  Port=2
  Compare To Zero : simulink/Logic and Bit Operations/Compare To Zero  relop=<=  OutDataTypeStr=boolean
  Multiport Switch2 : MultiPortSwitch  DataPortOrder=Zero-based contiguous  Inputs=2  zeroidx=on
  Subtract18 : Sum  Inputs=+-  OutDataTypeStr=fixdt(1,46,28)
  min : Outport
  wires:
  Subtract18/1 -> Compare To Zero/1
  b/1 -> Subtract18/2, Multiport Switch2/2
  a/1 -> Multiport Switch2/3, Subtract18/1
  Multiport Switch2/1 -> min/1
  Compare To Zero/1 -> Multiport Switch2/1

== system lib_rfsoc_fec/Soft Demodulation/Soft Demodulation/Subsystem1/get_min7 ==
  a : Inport
  b : Inport  Port=2
  Compare To Zero : simulink/Logic and Bit Operations/Compare To Zero  relop=<=  OutDataTypeStr=boolean
  Multiport Switch2 : MultiPortSwitch  DataPortOrder=Zero-based contiguous  Inputs=2  zeroidx=on
  Subtract18 : Sum  Inputs=+-  OutDataTypeStr=fixdt(1,46,28)
  min : Outport
  wires:
  Subtract18/1 -> Compare To Zero/1
  b/1 -> Subtract18/2, Multiport Switch2/2
  a/1 -> Multiport Switch2/3, Subtract18/1
  Multiport Switch2/1 -> min/1
  Compare To Zero/1 -> Multiport Switch2/1

== system lib_rfsoc_fec/Soft Demodulation/Soft Demodulation/Subsystem6/get_min1 ==
  a : Inport
  b : Inport  Port=2
  Compare To Zero : simulink/Logic and Bit Operations/Compare To Zero  relop=<=  OutDataTypeStr=boolean
  Multiport Switch2 : MultiPortSwitch  DataPortOrder=Zero-based contiguous  Inputs=2  zeroidx=on
  Subtract18 : Sum  Inputs=+-  OutDataTypeStr=fixdt(1,46,28)
  min : Outport
  wires:
  Subtract18/1 -> Compare To Zero/1
  b/1 -> Subtract18/2, Multiport Switch2/2
  a/1 -> Multiport Switch2/3, Subtract18/1
  Multiport Switch2/1 -> min/1
  Compare To Zero/1 -> Multiport Switch2/1

== system lib_rfsoc_fec/Soft Demodulation/Soft Demodulation/Subsystem6/get_min2 ==
  a : Inport
  b : Inport  Port=2
  Compare To Zero : simulink/Logic and Bit Operations/Compare To Zero  relop=<=  OutDataTypeStr=boolean
  Multiport Switch2 : MultiPortSwitch  DataPortOrder=Zero-based contiguous  Inputs=2  zeroidx=on
  Subtract18 : Sum  Inputs=+-  OutDataTypeStr=fixdt(1,46,28)
  min : Outport
  wires:
  Compare To Zero/1 -> Multiport Switch2/1
  Multiport Switch2/1 -> min/1
  a/1 -> Subtract18/1, Multiport Switch2/3
  b/1 -> Multiport Switch2/2, Subtract18/2
  Subtract18/1 -> Compare To Zero/1

== system lib_rfsoc_fec/Soft Demodulation/Soft Demodulation/Subsystem6/get_min3 ==
  a : Inport
  b : Inport  Port=2
  Compare To Zero : simulink/Logic and Bit Operations/Compare To Zero  relop=<=  OutDataTypeStr=boolean
  Multiport Switch2 : MultiPortSwitch  DataPortOrder=Zero-based contiguous  Inputs=2  zeroidx=on
  Subtract18 : Sum  Inputs=+-  OutDataTypeStr=fixdt(1,46,28)
  min : Outport
  wires:
  Subtract18/1 -> Compare To Zero/1
  b/1 -> Subtract18/2, Multiport Switch2/2
  a/1 -> Multiport Switch2/3, Subtract18/1
  Multiport Switch2/1 -> min/1
  Compare To Zero/1 -> Multiport Switch2/1

== system lib_rfsoc_fec/Soft Demodulation/Soft Demodulation/Subsystem6/get_min4 ==
  a : Inport
  b : Inport  Port=2
  Compare To Zero : simulink/Logic and Bit Operations/Compare To Zero  relop=<=  OutDataTypeStr=boolean
  Multiport Switch2 : MultiPortSwitch  DataPortOrder=Zero-based contiguous  Inputs=2  zeroidx=on
  Subtract18 : Sum  Inputs=+-  OutDataTypeStr=fixdt(1,46,28)
  min : Outport
  wires:
  Compare To Zero/1 -> Multiport Switch2/1
  Multiport Switch2/1 -> min/1
  a/1 -> Subtract18/1, Multiport Switch2/3
  b/1 -> Multiport Switch2/2, Subtract18/2
  Subtract18/1 -> Compare To Zero/1

== system lib_rfsoc_fec/Soft Demodulation/Soft Demodulation/Subsystem6/get_min5 ==
  a : Inport
  b : Inport  Port=2
  Compare To Zero : simulink/Logic and Bit Operations/Compare To Zero  relop=<=  OutDataTypeStr=boolean
  Multiport Switch2 : MultiPortSwitch  DataPortOrder=Zero-based contiguous  Inputs=2  zeroidx=on
  Subtract18 : Sum  Inputs=+-  OutDataTypeStr=fixdt(1,46,28)
  min : Outport
  wires:
  Subtract18/1 -> Compare To Zero/1
  b/1 -> Subtract18/2, Multiport Switch2/2
  a/1 -> Multiport Switch2/3, Subtract18/1
  Multiport Switch2/1 -> min/1
  Compare To Zero/1 -> Multiport Switch2/1

== system lib_rfsoc_fec/Soft Demodulation/Soft Demodulation/Subsystem6/get_min6 ==
  a : Inport
  b : Inport  Port=2
  Compare To Zero : simulink/Logic and Bit Operations/Compare To Zero  relop=<=  OutDataTypeStr=boolean
  Multiport Switch2 : MultiPortSwitch  DataPortOrder=Zero-based contiguous  Inputs=2  zeroidx=on
  Subtract18 : Sum  Inputs=+-  OutDataTypeStr=fixdt(1,46,28)
  min : Outport
  wires:
  Compare To Zero/1 -> Multiport Switch2/1
  Multiport Switch2/1 -> min/1
  a/1 -> Subtract18/1, Multiport Switch2/3
  b/1 -> Multiport Switch2/2, Subtract18/2
  Subtract18/1 -> Compare To Zero/1

== system lib_rfsoc_fec/Soft Demodulation/Soft Demodulation/Subsystem6/get_min7 ==
  a : Inport
  b : Inport  Port=2
  Compare To Zero : simulink/Logic and Bit Operations/Compare To Zero  relop=<=  OutDataTypeStr=boolean
  Multiport Switch2 : MultiPortSwitch  DataPortOrder=Zero-based contiguous  Inputs=2  zeroidx=on
  Subtract18 : Sum  Inputs=+-  OutDataTypeStr=fixdt(1,46,28)
  min : Outport
  wires:
  Compare To Zero/1 -> Multiport Switch2/1
  Multiport Switch2/1 -> min/1
  a/1 -> Subtract18/1, Multiport Switch2/3
  b/1 -> Multiport Switch2/2, Subtract18/2
  Subtract18/1 -> Compare To Zero/1

== matlab function lib_rfsoc_fec/Soft Demodulation/symmetric_saturation ==
  data: u input; y output
function y = symmetric_saturation(u)
    if u > 7.75
        y = fi(7.75, 1, 6, 2);
    elseif u < -7.75
        y = fi(-7.75, 1, 6, 2);
    else
        y = fi(u, 1, 6, 2);
    end

== matlab function lib_rfsoc_fec/Soft Demodulation/MATLAB Function ==
  data: u input; y output; reset input
function y = max_magnitude(u, reset)
    persistent max
    
    if isempty(max)
        max = fi(0, 0, 32, 24);
    end

   if abs(u) > max
       max(:) = abs(u);
   end
   
   if reset
       max(:) = 0;
   end
   
   y = fi(max, 0, 32, 24);
    
end

== stateflow chart lib_rfsoc_fec/FEC Ctrl/Chart ==
  settings: executeAtInitialization=1
  state IDLE
    % Local
    %
    % DATA Stream
    m_axis_tvalid(:) = false;
    m_axis_lane0_tdata(:) = 0;
    m_axis_lane1_tdata(:) = 0;
    m_axis_lane2_tdata(:) = 0;
    m_axis_lane3_tdata(:) = 0;
    %
    % CTRL Stream
    m_axis_ctrl_tdata = fi(0,0,32,0);
    m_axis_ctrl_tlast = false;
    m_axis_ctrl_tvalid = false;
    %
    % STATUS Stream
    s_axis_status_tready = false;
  state LOAD_NVALID
    % Local
    loaded_n(:) = block_length;
    loaded_ctrl(:) = ctrl_word;
    %
    % DATA Stream
    m_axis_tvalid(:) = false;
    m_axis_lane0_tdata(:) = 0;
    m_axis_lane1_tdata(:) = 0;
    m_axis_lane2_tdata(:) = 0;
    m_axis_lane3_tdata(:) = 0;
    %
    % CTRL Stream
    m_axis_ctrl_tdata(:) = 0;
    m_axis_ctrl_tlast(:) = false;
    m_axis_ctrl_tvalid(:) = false;
    %
    % STATUS Stream
    s_axis_status_tready(:) = true;
  state LOAD_VALID
    % Local
    count(:) = count + 1;
    loaded_n(:) = block_length;
    loaded_ctrl(:) = ctrl_word;
    %
    % DATA Stream
    m_axis_tvalid(:) = true;
    m_axis_lane0_tdata(:) = s_axis_lane0_tdata;
    m_axis_lane1_tdata(:) = s_axis_lane1_tdata;
    m_axis_lane2_tdata(:) = s_axis_lane2_tdata;
    m_axis_lane3_tdata(:) = s_axis_lane3_tdata;
    %
    % CTRL Stream
    m_axis_ctrl_tdata(:) = 0;
    m_axis_ctrl_tlast(:) = false;
    m_axis_ctrl_tvalid(:) = false;
    %
    % STATUS Stream
    s_axis_status_tready(:) = true;
  state INIT
    % Local
    count = fi(0,0,32,0);
    n = fi(0,0,32,0);
    loaded_n = fi(0,0,32,0);
    loaded_ctrl = fi(0,0,32,0);
    %
    % DATA Stream
    m_axis_tvalid = false;
    m_axis_lane0_tdata = fi(0,0,128,0);
    m_axis_lane1_tdata = fi(0,0,128,0);
    m_axis_lane2_tdata = fi(0,0,128,0);
    m_axis_lane3_tdata = fi(0,0,128,0);
    %
    % CTRL Stream
    m_axis_ctrl_tdata = fi(0,0,32,0);
    m_axis_ctrl_tlast = false;
    m_axis_ctrl_tvalid = false;
    %
    % STATUS Stream
    s_axis_status_tready = false;
  state COUNT_DIN
    % Local
    count(:) = count + 1;
    %
    % DATA Stream
    m_axis_tvalid(:) = true;
    m_axis_lane0_tdata(:) = s_axis_lane0_tdata;
    m_axis_lane1_tdata(:) = s_axis_lane1_tdata;
    m_axis_lane2_tdata(:) = s_axis_lane2_tdata;
    m_axis_lane3_tdata(:) = s_axis_lane3_tdata;        % Complete a full block
    %
    % CTRL Stream
    m_axis_ctrl_tdata(:) = 0;
    m_axis_ctrl_tlast(:) = false;
    m_axis_ctrl_tvalid(:) = false;
    %
    % STATUS Stream
    s_axis_status_tready(:) = true;
  state CTRL
    % Local
    count(:) = count + 1;
    n(:) = loaded_n;
    %
    % DATA Stream
    m_axis_tvalid(:) = true;
    m_axis_lane0_tdata(:) = s_axis_lane0_tdata;
    m_axis_lane1_tdata(:) = s_axis_lane1_tdata;
    m_axis_lane2_tdata(:) = s_axis_lane2_tdata;
    m_axis_lane3_tdata(:) = s_axis_lane3_tdata;
    %
    % CTRL Stream
    m_axis_ctrl_tdata(:) = loaded_ctrl;
    m_axis_ctrl_tlast(:) = true;
    m_axis_ctrl_tvalid(:) = true;
    %
    % STATUS Stream
    s_axis_status_tready(:) = true;
  state WAITING
    % Local
    %
    % DATA Stream
    m_axis_tvalid(:) = false;
    m_axis_lane0_tdata(:) = s_axis_lane0_tdata;
    m_axis_lane1_tdata(:) = s_axis_lane1_tdata;
    m_axis_lane2_tdata(:) = s_axis_lane2_tdata;
    m_axis_lane3_tdata(:) = s_axis_lane3_tdata;
    %
    % CTRL Stream
    m_axis_ctrl_tdata(:) = 0;
    m_axis_ctrl_tlast(:) = false;
    m_axis_ctrl_tvalid(:) = false;
    %
    % STATUS Stream
    s_axis_status_tready(:) = true;
  LOAD_VALID -> IDLE [order 3] : [count >= n && s_axis_tvalid == 0]{count(:) = 0}
  (default) -> INIT
  LOAD_NVALID -> COUNT_DIN [order 2] : [s_axis_tvalid == 1 && count > 0]
  LOAD_VALID -> CTRL [order 2] : [count >= n && s_axis_tvalid == 1]{count(:) = 0}
  IDLE -> LOAD_NVALID [order 1] : [load == 1]
  INIT -> IDLE
  LOAD_VALID -> COUNT_DIN [order 1] : [count < n]
  CTRL -> LOAD_VALID [order 1] : [load == 1 && s_axis_tvalid == 1]
  COUNT_DIN -> LOAD_NVALID [order 5] : [load == 1 && s_axis_tvalid == 0]
  LOAD_NVALID -> CTRL [order 1] : [s_axis_tvalid == 1 && count ==0]
  COUNT_DIN -> IDLE [order 3] : [count >= n && s_axis_tvalid == 0]{count(:) = 0}
  IDLE -> CTRL [order 2] : [s_axis_tvalid == 1 && count ==0]
  COUNT_DIN -> LOAD_VALID [order 2] : [load == 1 && s_axis_tvalid == 1]
  COUNT_DIN -> WAITING [order 4] : [load == 0 && s_axis_tvalid == 0]
  CTRL -> COUNT_DIN [order 2] : [s_axis_tvalid == 1]
  COUNT_DIN -> CTRL [order 1] : [count >= n && s_axis_tvalid == 1]{count(:) = 0}
  WAITING -> COUNT_DIN : [s_axis_tvalid == 1]
  CTRL -> WAITING [order 3] : [s_axis_tvalid == 0]
  data: m_axis_ctrl_tvalid output; ctrl_word input; count local; m_axis_ctrl_tdata output; m_axis_ctrl_tlast output; m_axis_tvalid output; block_length input; load input; s_axis_tvalid input; s_axis_status_tready output; n local; loaded_ctrl local; loaded_n local; state output Enum: stateType; m_axis_lane0_tdata output; m_axis_lane1_tdata output; m_axis_lane2_tdata output; m_axis_lane3_tdata output; s_axis_lane1_tdata input; s_axis_lane2_tdata input; s_axis_lane3_tdata input; s_axis_lane0_tdata input
